simulink model "TemplateNoLineal2_2015b"  (R2023b)
settings: Solver=ode4  StartTime=0.0  StopTime=10.0  FixedStep=0.0001  RelTol=1e-3
undefined symbols (not defined in the file): ue, x1e, x2e
libraries: cstblocks x1
settings Model: Creator=aghersin  LastModifiedBy=Usuario
settings SolverCC: AlgebraicLoopSolver=TrustRegion
settings DataIOCC: ReturnWorkspaceOutputs=off
settings OptimizationCC: LifeSpan=inf
settings DebuggingCC: UnconnectedInputMsg=warning  UnconnectedOutputMsg=warning  UnconnectedLineMsg=warning  SFExecutionAtInitializationDiag=none  ArithmeticOperatorsInVariantConditions=warning
settings ModelReferenceCC: EnableRefExpFcnMdlSchedulingChecks=on
settings SFSimCC: SimUseLocalCustomCode=off  CustomCodeUndefinedFunction=UseInterfaceOnly
settings RTWCC: RTWUseLocalCustomCode=off
settings CodeAppCC: StateflowObjectComments=on

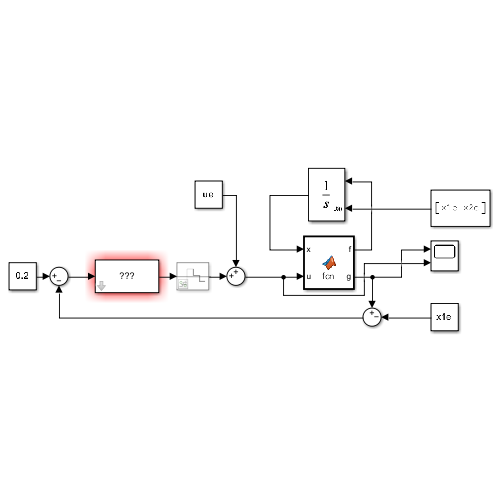
[thumbnail: Simulink's stored preview of the top-level diagram]
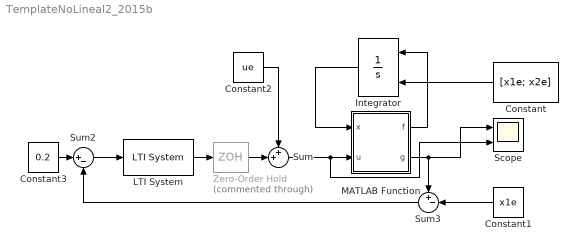
== system TemplateNoLineal2_2015b ==
  Constant : Constant  Value=[x1e; x2e]
  Constant1 : Constant  Value=x1e
  Constant2 : Constant  Value=ue
  Constant3 : Constant  Value=0.2
  Integrator : Integrator  InitialConditionSource=external
  LTI System : cstblocks/LTI System  sys=C_discretizado  IC=[]  PadeOrder=0
  MATLAB Function : MATLAB Function  TreatAsAtomicUnit=on
  Scope : Scope  NumInputPorts=2
  Sum : Sum  Inputs=++|
  Sum2 : Sum  Inputs=|+-
  Sum3 : Sum  Inputs=+-|
  Zero-Order Hold : ZeroOrderHold  Commented=through  SampleTime=0.28
  wires:
  Integrator/1 -> MATLAB Function/1(x)
  MATLAB Function/1(f) -> Integrator/1
  Constant/1 -> Integrator/2
  MATLAB Function/2(g) -> Sum3/1, Scope/1
  Constant1/1 -> Sum3/2
  Constant2/1 -> Sum/1
  Sum2/1 -> LTI System/1
  Constant3/1 -> Sum2/1
  Sum3/1 -> Sum2/2
  LTI System/1 -> Zero-Order Hold/1
  Sum/1 -> Scope/2, MATLAB Function/2(u)
  Zero-Order Hold/1 -> Sum/2

== matlab function TemplateNoLineal2_2015b/MATLAB Function ==
  data: x input; u input; f output; g output
function [f, g] = fcn(x,u)

f1 = x(2);
f2 = u - sin(x(1));
f = [f1; f2];

g = x(1);
